simulink model "ivedsp"  (Simulink 7.6)
settings: Solver=FixedStepDiscrete  StartTime=0.0  StopTime=10  FixedStep=1  RelTol=1e-3
libraries: simulink x42
settings Model: Creator=jordan  LastModifiedBy=jordan
settings DataIOCC: LimitDataPoints=off  SaveOutput=off  SignalLogging=off  DSMLogging=off  SaveTime=off
settings OptimizationCC: BlockReduction=off  ConditionallyExecuteInputs=off  InlineParams=on

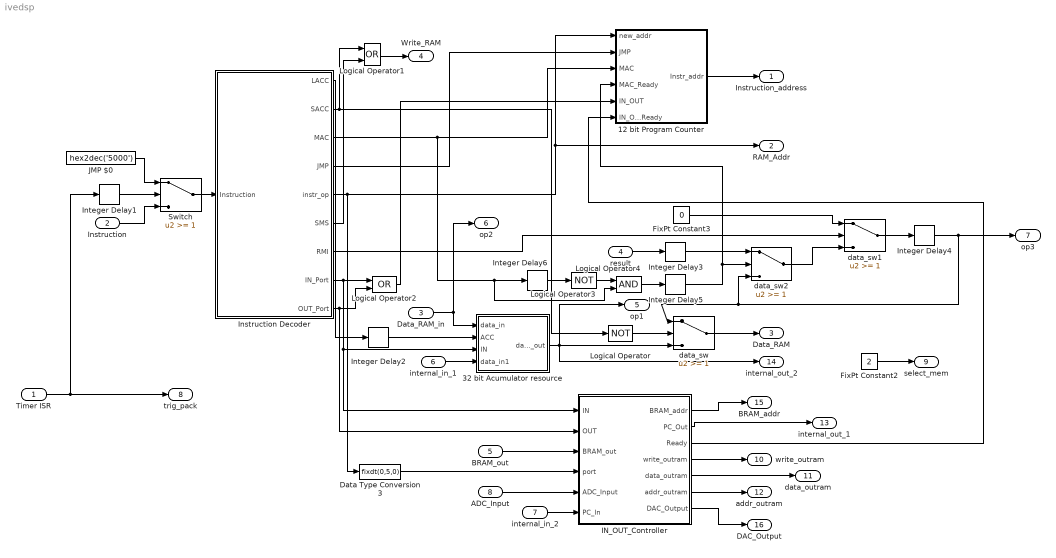
== system ivedsp ==
  Timer ISR : Inport  OutDataTypeStr=boolean
  Instruction : Inport  Port=2  OutDataTypeStr=uint16
  Data_RAM_in : Inport  Port=3  OutDataTypeStr=uint32
  result : Inport  Port=4  OutDataTypeStr=uint32
  BRAM_out : Inport  Port=5  OutDataTypeStr=uint8
  internal_in_1 : Inport  Port=6  OutDataTypeStr=uint32
  internal_in_2 : Inport  Port=7  OutDataTypeStr=uint8  PortDimensions=4
  ADC_Input : Inport  Port=8  OutDataTypeStr=uint8  PortDimensions=8
  12 bit Program Counter : Subsystem
  32 bit Acumulator resource : Subsystem
  Data Type Conversion3 : DataTypeConversion  OutDataTypeStr=fixdt(0,5,0)
  FixPt Constant2 : Constant  DisableCoverage=on  Value=2  OutDataTypeStr=fixdt(0,4,0)
  FixPt Constant3 : Constant  DisableCoverage=on  Value=0  OutDataTypeStr=uint32
  IN_OUT_Controller : Subsystem
  Instruction Decoder : Subsystem
  Integer Delay{1..4,6} (5 alike) : simulink/Discrete/Integer Delay  NumDelays=1  vinit=0.0  samptime=-1
  Integer Delay5 : simulink/Discrete/Integer Delay  NumDelays=3  vinit=0.0  samptime=-1
  JMP $0 : Constant  DisableCoverage=on  Value=hex2dec('5000')  OutDataTypeStr=Inherit: Inherit via back propagation
  Logical Operator : Logic  Operator=NOT  AllPortsSameDT=off  OutDataTypeStr=boolean
  Logical Operator1 : Logic  Operator=OR  AllPortsSameDT=off  OutDataTypeStr=boolean
  Logical Operator2 : Logic  Operator=OR  AllPortsSameDT=off  OutDataTypeStr=boolean
  Logical Operator3 : Logic  Operator=NOT  AllPortsSameDT=off  OutDataTypeStr=boolean
  Logical Operator4 : Logic  AllPortsSameDT=off  OutDataTypeStr=boolean
  Switch : Switch  Threshold=1
  data_sw : Switch  Threshold=1
  data_sw1 : Switch  Threshold=1
  data_sw2 : Switch  Threshold=1
  Instruction_address : Outport  OutDataTypeStr=fixdt(0,12,0)
  RAM_Addr : Outport  Port=2  OutDataTypeStr=fixdt(0,12,0)
  Data_RAM : Outport  Port=3  OutDataTypeStr=uint32
  Write_RAM : Outport  Port=4  OutDataTypeStr=boolean
  op1 : Outport  Port=5  OutDataTypeStr=uint32
  op2 : Outport  Port=6  OutDataTypeStr=uint32
  op3 : Outport  Port=7  OutDataTypeStr=uint32
  trig_pack : Outport  Port=8
  select_mem : Outport  Port=9
  write_outram : Outport  Port=10  OutDataTypeStr=boolean
  data_outram : Outport  Port=11  OutDataTypeStr=uint8
  addr_outram : Outport  Port=12  OutDataTypeStr=fixdt(0,14,0)
  internal_out_1 : Outport  Port=13
  internal_out_2 : Outport  Port=14  OutDataTypeStr=uint32
  BRAM_addr : Outport  Port=15
  DAC_Output : Outport  Port=16
  wires:
  32 bit Acumulator resource/1(data_out) -> data_sw/3, op1/1, internal_out_2/1
  Data_RAM_in/1 -> 32 bit Acumulator resource/1(data_in), op2/1
  Instruction Decoder/5(instr_op) -> 12 bit Program Counter/1(new_addr), RAM_Addr/1, Data Type Conversion3/1
  Instruction Decoder/1(LACC) -> Integer Delay2/1
  Integer Delay2/1 -> 32 bit Acumulator resource/2(ACC)
  Instruction Decoder/2(SACC) -> Logical Operator/1, Logical Operator1/1
  Logical Operator/1 -> data_sw/2
  Instruction Decoder/4(JMP) -> 12 bit Program Counter/2(JMP)
  Instruction Decoder/3(MAC) -> 12 bit Program Counter/3(MAC), Logical Operator4/2, Integer Delay6/1
  Instruction Decoder/7(RMI) -> data_sw1/2
  Instruction Decoder/6(SMS) -> Logical Operator1/2
  Instruction Decoder/8(IN_Port) -> 32 bit Acumulator resource/3(IN), IN_OUT_Controller/1(IN), Logical Operator2/1
  Data Type Conversion3/1 -> IN_OUT_Controller/4(port)
  Switch/1 -> Instruction Decoder/1(Instruction)
  JMP $0/1 -> Switch/1
  12 bit Program Counter/1(Instr_addr) -> Instruction_address/1
  Instruction/1 -> Switch/3
  data_sw/1 -> Data_RAM/1
  Logical Operator1/1 -> Write_RAM/1
  result/1 -> Integer Delay3/1
  Instruction Decoder/9(OUT_Port) -> Logical Operator2/2, IN_OUT_Controller/2(OUT)
  IN_OUT_Controller/6(addr_outram) -> addr_outram/1
  IN_OUT_Controller/4(write_outram) -> write_outram/1
  IN_OUT_Controller/5(data_outram) -> data_outram/1
  Logical Operator2/1 -> 12 bit Program Counter/5(IN_OUT)
  internal_in_1/1 -> 32 bit Acumulator resource/4(data_in1)
  internal_in_2/1 -> IN_OUT_Controller/6(PC_In)
  Integer Delay1/1 -> Switch/2
  FixPt Constant2/1 -> select_mem/1
  Timer ISR/1 -> trig_pack/1, Integer Delay1/1
  Integer Delay4/1 -> op3/1, data_sw2/3, data_sw/1
  data_sw1/1 -> Integer Delay4/1
  FixPt Constant3/1 -> data_sw1/1
  data_sw2/1 -> data_sw1/3
  Integer Delay3/1 -> data_sw2/1
  Integer Delay5/1 -> 12 bit Program Counter/4(MAC_Ready), data_sw2/2
  Integer Delay6/1 -> Logical Operator3/1
  Logical Operator3/1 -> Logical Operator4/1
  Logical Operator4/1 -> Integer Delay5/1
  IN_OUT_Controller/7(DAC_Output) -> DAC_Output/1
  IN_OUT_Controller/3(Ready) -> 12 bit Program Counter/6(IN_OUT_Ready)
  BRAM_out/1 -> IN_OUT_Controller/3(BRAM_out)
  ADC_Input/1 -> IN_OUT_Controller/5(ADC_Input)
  IN_OUT_Controller/2(PC_Out) -> internal_out_1/1
  IN_OUT_Controller/1(BRAM_addr) -> BRAM_addr/1

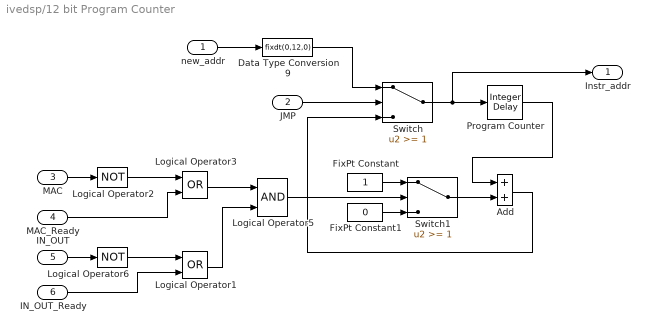
== system ivedsp/12 bit Program Counter ==
  new_addr : Inport
  JMP : Inport  Port=2
  MAC : Inport  Port=3  OutDataTypeStr=boolean
  MAC_Ready : Inport  Port=4  OutDataTypeStr=boolean
  IN_OUT : Inport  Port=5  OutDataTypeStr=boolean
  IN_OUT_Ready : Inport  Port=6  OutDataTypeStr=boolean
  Add : Sum  AccumDataTypeStr=fixdt(0,12,0)  OutDataTypeStr=fixdt(0,12,0)
  Data Type Conversion9 : DataTypeConversion  OutDataTypeStr=fixdt(0,12,0)
  FixPt Constant : Constant  DisableCoverage=on  OutDataTypeStr=fixdt(0,12,0)
  FixPt Constant1 : Constant  DisableCoverage=on  Value=0  OutDataTypeStr=fixdt(0,12,0)
  Logical Operator1 : Logic  Operator=OR  AllPortsSameDT=off  OutDataTypeStr=boolean
  Logical Operator2 : Logic  Operator=NOT  AllPortsSameDT=off  OutDataTypeStr=boolean
  Logical Operator3 : Logic  Operator=OR  AllPortsSameDT=off  OutDataTypeStr=boolean
  Logical Operator5 : Logic  AllPortsSameDT=off  OutDataTypeStr=boolean
  Logical Operator6 : Logic  Operator=NOT  AllPortsSameDT=off  OutDataTypeStr=boolean
  Program Counter : simulink/Discrete/Integer Delay  NumDelays=1  vinit=0.0  samptime=-1
  Switch : Switch  Threshold=1
  Switch1 : Switch  Threshold=1
  Instr_addr : Outport  InitialOutput=0
  wires:
  JMP/1 -> Switch/2
  new_addr/1 -> Data Type Conversion9/1
  Program Counter/1 -> Add/1
  Switch/1 -> Program Counter/1, Instr_addr/1
  FixPt Constant/1 -> Switch1/1
  Add/1 -> Switch/3
  Data Type Conversion9/1 -> Switch/1
  Switch1/1 -> Add/2
  FixPt Constant1/1 -> Switch1/3
  Logical Operator3/1 -> Logical Operator5/1
  Logical Operator2/1 -> Logical Operator3/1
  MAC/1 -> Logical Operator2/1
  Logical Operator1/1 -> Logical Operator5/2
  Logical Operator6/1 -> Logical Operator1/1
  IN_OUT/1 -> Logical Operator6/1
  IN_OUT_Ready/1 -> Logical Operator1/2
  Logical Operator5/1 -> Switch1/2
  MAC_Ready/1 -> Logical Operator3/2

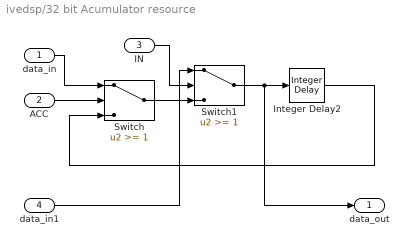
== system ivedsp/32 bit Acumulator resource ==
  data_in : Inport
  ACC : Inport  Port=2
  IN : Inport  Port=3
  data_in1 : Inport  Port=4
  Integer Delay2 : simulink/Discrete/Integer Delay  NumDelays=1  vinit=0.0  samptime=-1
  Switch : Switch  Threshold=1
  Switch1 : Switch  Threshold=1
  data_out : Outport  OutDataTypeStr=uint32
  wires:
  Switch/1 -> Switch1/3
  Integer Delay2/1 -> Switch/3
  data_in/1 -> Switch/1
  ACC/1 -> Switch/2
  Switch1/1 -> Integer Delay2/1, data_out/1
  IN/1 -> Switch1/2
  data_in1/1 -> Switch1/1

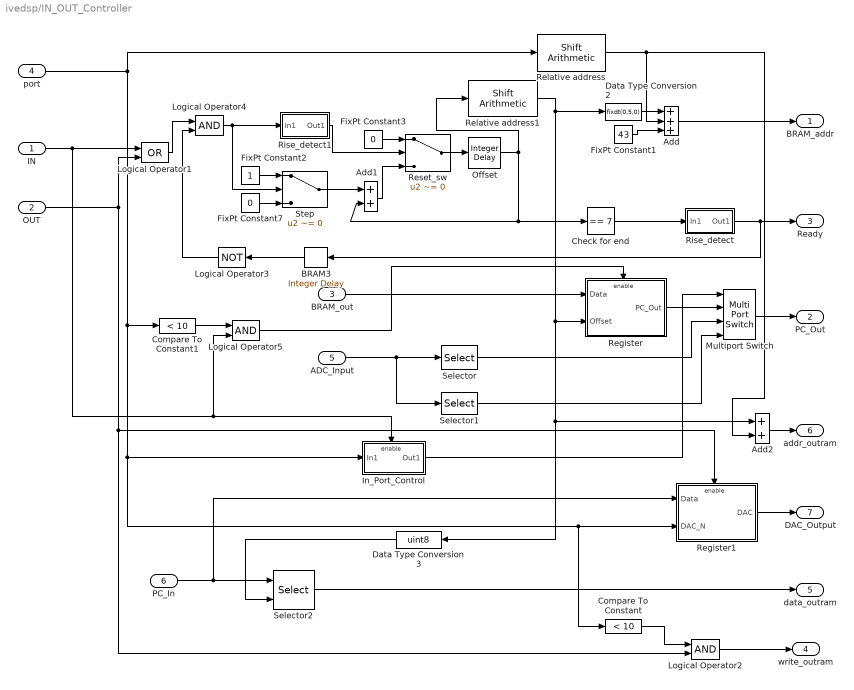
== system ivedsp/IN_OUT_Controller ==
  IN : Inport  OutDataTypeStr=boolean
  OUT : Inport  Port=2  OutDataTypeStr=boolean
  BRAM_out : Inport  Port=3  OutDataTypeStr=uint8
  port : Inport  Port=4  OutDataTypeStr=fixdt(0,5,0)
  ADC_Input : Inport  Port=5  OutDataTypeStr=uint8  PortDimensions=8
  PC_In : Inport  Port=6  OutDataTypeStr=uint8  PortDimensions=4
  Add : Sum  Inputs=+++  AccumDataTypeStr=fixdt(0,11,0)  OutDataTypeStr=fixdt(0,11,0)  SaturateOnIntegerOverflow=on
  Add1 : Sum  AccumDataTypeStr=fixdt(0,3,0)  OutDataTypeStr=fixdt(0,3,0)  SaturateOnIntegerOverflow=on
  Add2 : Sum  AccumDataTypeStr=fixdt(0,14,0)  OutDataTypeStr=fixdt(0,14,0)
  BRAM3 : simulink/Discrete/Integer Delay  NumDelays=1  vinit=0.0  samptime=-1
  Check for end : simulink/Logic and Bit Operations/Compare To Constant  SystemSampleTime=-1  relop===  const=7  LogicOutDataTypeMode=boolean
  Compare To Constant : simulink/Logic and Bit Operations/Compare To Constant  SystemSampleTime=-1  relop=<  const=10  LogicOutDataTypeMode=boolean
  Compare To Constant1 : simulink/Logic and Bit Operations/Compare To Constant  SystemSampleTime=-1  relop=<  const=10  LogicOutDataTypeMode=boolean
  Data Type Conversion2 : DataTypeConversion  OutDataTypeStr=fixdt(0,5,0)
  Data Type Conversion3 : DataTypeConversion  OutDataTypeStr=uint8
  FixPt Constant1 : Constant  DisableCoverage=on  Value=43  OutDataTypeStr=fixdt(0,11,0)
  FixPt Constant2 : Constant  DisableCoverage=on  OutDataTypeStr=fixdt(0,3,0)
  FixPt Constant3 : Constant  DisableCoverage=on  Value=0  OutDataTypeStr=fixdt(0,3,0)
  FixPt Constant7 : Constant  DisableCoverage=on  Value=0  OutDataTypeStr=fixdt(0,3,0)
  In_Port_Control : Subsystem
  Logical Operator1 : Logic  Operator=OR  AllPortsSameDT=off  OutDataTypeStr=boolean
  Logical Operator2 : Logic  AllPortsSameDT=off  OutDataTypeStr=boolean
  Logical Operator3 : Logic  Operator=NOT  AllPortsSameDT=off  OutDataTypeStr=boolean
  Logical Operator4 : Logic  AllPortsSameDT=off  OutDataTypeStr=boolean
  Logical Operator5 : Logic  AllPortsSameDT=off  OutDataTypeStr=boolean
  Multiport Switch : MultiPortSwitch  DataPortOrder=Zero-based contiguous  zeroidx=on
  Offset : simulink/Discrete/Integer Delay  NumDelays=1  vinit=0.0  samptime=0
  Register : Subsystem
  Register1 : Subsystem
  Relative address : simulink/Logic and Bit Operations/Shift Arithmetic  SystemSampleTime=-1  nBitShiftRight=-2  nBinPtShiftRight=0
  Relative address1 : simulink/Logic and Bit Operations/Shift Arithmetic  SystemSampleTime=-1  nBitShiftRight=1  nBinPtShiftRight=0
  Reset_sw : Switch  Criteria=u2 ~= 0
  Rise_detect : Subsystem
  Rise_detect1 : Subsystem
  Selector : Selector  InputPortWidth=8  IndexOptions=Index vector (dialog)  Indices=1:4  OutputSizes=1
  Selector1 : Selector  InputPortWidth=8  IndexOptions=Index vector (dialog)  Indices=5:8  OutputSizes=1
  Selector2 : Selector  IndexMode=Zero-based  InputPortWidth=4  IndexOptions=Index vector (port)  Indices=5:8  OutputSizes=1
  Step : Switch  Criteria=u2 ~= 0
  BRAM_addr : Outport
  PC_Out : Outport  Port=2  OutDataTypeStr=uint8  PortDimensions=4
  Ready : Outport  Port=3
  write_outram : Outport  Port=4
  data_outram : Outport  Port=5
  addr_outram : Outport  Port=6
  DAC_Output : Outport  Port=7  OutDataTypeStr=uint8  PortDimensions=8
  wires:
  Register1/1(DAC) -> DAC_Output/1
  OUT/1 -> Logical Operator1/2, Logical Operator2/2, Register1/Enable
  IN/1 -> Logical Operator1/1, In_Port_Control/Enable, Logical Operator5/2
  Selector2/1 -> data_outram/1
  PC_In/1 -> Selector2/1, Register1/1(Data)
  Add2/1 -> addr_outram/1
  BRAM_out/1 -> Register/1(Data)
  FixPt Constant7/1 -> Step/3
  Step/1 -> Add1/1
  In_Port_Control/1(Out1) -> Multiport Switch/1
  Selector1/1 -> Multiport Switch/4
  ADC_Input/1 -> Selector1/1, Selector/1
  Selector/1 -> Multiport Switch/3
  Multiport Switch/1 -> PC_Out/1
  Check for end/1 -> Rise_detect/1(In1)
  FixPt Constant3/1 -> Reset_sw/1
  Rise_detect1/1(Out1) -> Reset_sw/2
  Register/1(PC_Out) -> Multiport Switch/2
  Logical Operator4/1 -> Rise_detect1/1(In1), Step/2
  port/1 -> Relative address/1, In_Port_Control/1(In1), Register1/2(DAC_N), Compare To Constant/1, Compare To Constant1/1
  Relative address/1 -> Add2/2, Add/2
  FixPt Constant2/1 -> Step/1
  Add1/1 -> Reset_sw/3
  Reset_sw/1 -> Offset/1
  FixPt Constant1/1 -> Add/3
  Data Type Conversion2/1 -> Add/1
  Add/1 -> BRAM_addr/1
  Offset/1 -> Relative address1/1, Add1/2, Check for end/1
  Rise_detect/1(Out1) -> Ready/1, BRAM3/1
  Data Type Conversion3/1 -> Selector2/2
  Relative address1/1 -> Data Type Conversion2/1, Register/2(Offset), Add2/1, Data Type Conversion3/1
  Logical Operator2/1 -> write_outram/1
  Compare To Constant/1 -> Logical Operator2/1
  Logical Operator3/1 -> Logical Operator4/2
  Logical Operator1/1 -> Logical Operator4/1
  BRAM3/1 -> Logical Operator3/1
  Logical Operator5/1 -> Register/Enable
  Compare To Constant1/1 -> Logical Operator5/1

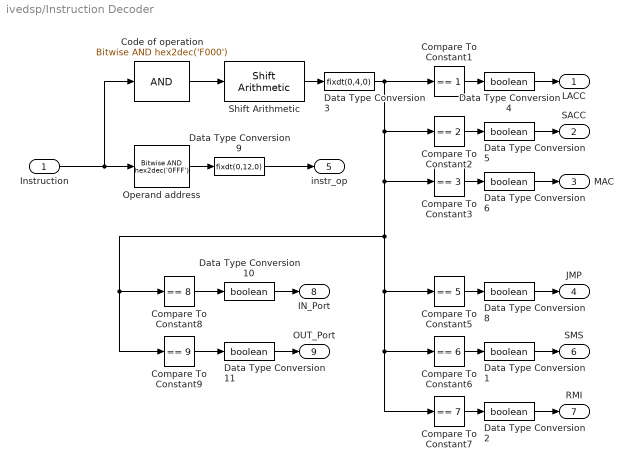
== system ivedsp/Instruction Decoder ==
  Instruction : Inport  OutDataTypeStr=uint16
  Code of operation : simulink/Logic and Bit Operations/Bitwise Operator  logicop=AND  UseBitMask=on  BitMask=hex2dec('F000')  BitMaskRealWorld=Stored Integer
  Compare To Constant1 : simulink/Logic and Bit Operations/Compare To Constant  SystemSampleTime=-1  relop===  const=1  LogicOutDataTypeMode=boolean
  Compare To Constant2 : simulink/Logic and Bit Operations/Compare To Constant  SystemSampleTime=-1  relop===  const=2  LogicOutDataTypeMode=boolean
  Compare To Constant3 : simulink/Logic and Bit Operations/Compare To Constant  SystemSampleTime=-1  relop===  const=3  LogicOutDataTypeMode=boolean
  Compare To Constant5 : simulink/Logic and Bit Operations/Compare To Constant  SystemSampleTime=-1  relop===  const=5  LogicOutDataTypeMode=boolean
  Compare To Constant6 : simulink/Logic and Bit Operations/Compare To Constant  SystemSampleTime=-1  relop===  const=6  LogicOutDataTypeMode=boolean
  Compare To Constant7 : simulink/Logic and Bit Operations/Compare To Constant  SystemSampleTime=-1  relop===  const=7  LogicOutDataTypeMode=boolean
  Compare To Constant8 : simulink/Logic and Bit Operations/Compare To Constant  SystemSampleTime=-1  relop===  const=8  LogicOutDataTypeMode=boolean
  Compare To Constant9 : simulink/Logic and Bit Operations/Compare To Constant  SystemSampleTime=-1  relop===  const=9  LogicOutDataTypeMode=boolean
  Data Type Conversion{1..2,4..6,8,10..11} (8 alike) : DataTypeConversion  OutDataTypeStr=boolean
  Data Type Conversion3 : DataTypeConversion  OutDataTypeStr=fixdt(0,4,0)
  Data Type Conversion9 : DataTypeConversion  OutDataTypeStr=fixdt(0,12,0)
  Operand address : simulink/Logic and Bit Operations/Bitwise Operator  logicop=AND  UseBitMask=on  BitMask=hex2dec('0FFF')  BitMaskRealWorld=Stored Integer
  Shift Arithmetic : simulink/Logic and Bit Operations/Shift Arithmetic  SystemSampleTime=-1  nBitShiftRight=12  nBinPtShiftRight=0
  LACC : Outport
  SACC : Outport  Port=2
  MAC : Outport  Port=3
  JMP : Outport  Port=4
  instr_op : Outport  Port=5
  SMS : Outport  Port=6
  RMI : Outport  Port=7
  IN_Port : Outport  Port=8
  OUT_Port : Outport  Port=9
  wires:
  Instruction/1 -> Operand address/1, Code of operation/1
  Code of operation/1 -> Shift Arithmetic/1
  Shift Arithmetic/1 -> Data Type Conversion3/1
  Data Type Conversion3/1 -> Compare To Constant6/1, Compare To Constant7/1, Compare To Constant5/1, Compare To Constant8/1, Compare To Constant9/1, Compare To Constant3/1, Compare To Constant2/1, Compare To Constant1/1
  Compare To Constant1/1 -> Data Type Conversion4/1
  Compare To Constant2/1 -> Data Type Conversion5/1
  Compare To Constant3/1 -> Data Type Conversion6/1
  Compare To Constant5/1 -> Data Type Conversion8/1
  Operand address/1 -> Data Type Conversion9/1
  Data Type Conversion4/1 -> LACC/1
  Data Type Conversion5/1 -> SACC/1
  Data Type Conversion9/1 -> instr_op/1
  Data Type Conversion6/1 -> MAC/1
  Data Type Conversion8/1 -> JMP/1
  Compare To Constant6/1 -> Data Type Conversion1/1
  Data Type Conversion1/1 -> SMS/1
  Compare To Constant7/1 -> Data Type Conversion2/1
  Data Type Conversion2/1 -> RMI/1
  Compare To Constant8/1 -> Data Type Conversion10/1
  Data Type Conversion10/1 -> IN_Port/1
  Compare To Constant9/1 -> Data Type Conversion11/1
  Data Type Conversion11/1 -> OUT_Port/1

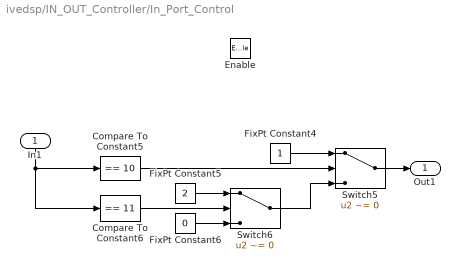
== system ivedsp/IN_OUT_Controller/In_Port_Control ==
  In1 : Inport
  Enable : EnablePort
  Compare To Constant5 : simulink/Logic and Bit Operations/Compare To Constant  SystemSampleTime=-1  relop===  const=10  LogicOutDataTypeMode=boolean
  Compare To Constant6 : simulink/Logic and Bit Operations/Compare To Constant  SystemSampleTime=-1  relop===  const=11  LogicOutDataTypeMode=boolean
  FixPt Constant4 : Constant  DisableCoverage=on  OutDataTypeStr=fixdt(0,2,0)
  FixPt Constant5 : Constant  DisableCoverage=on  Value=2  OutDataTypeStr=fixdt(0,2,0)
  FixPt Constant6 : Constant  DisableCoverage=on  Value=0  OutDataTypeStr=fixdt(0,2,0)
  Switch5 : Switch  Criteria=u2 ~= 0
  Switch6 : Switch  Criteria=u2 ~= 0
  Out1 : Outport  InitialOutput=0
  wires:
  Switch6/1 -> Switch5/3
  FixPt Constant6/1 -> Switch6/3
  FixPt Constant5/1 -> Switch6/1
  FixPt Constant4/1 -> Switch5/1
  Compare To Constant6/1 -> Switch6/2
  Compare To Constant5/1 -> Switch5/2
  In1/1 -> Compare To Constant6/1, Compare To Constant5/1
  Switch5/1 -> Out1/1

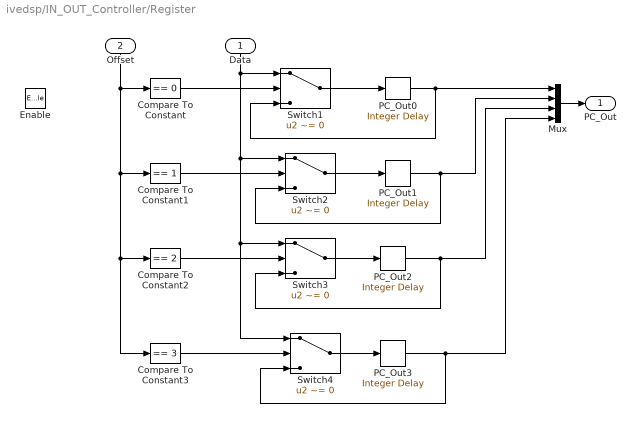
== system ivedsp/IN_OUT_Controller/Register ==
  Data : Inport
  Offset : Inport  Port=2
  Enable : EnablePort
  Compare To Constant : simulink/Logic and Bit Operations/Compare To Constant  SystemSampleTime=-1  relop===  const=0  LogicOutDataTypeMode=boolean
  Compare To Constant1 : simulink/Logic and Bit Operations/Compare To Constant  SystemSampleTime=-1  relop===  const=1  LogicOutDataTypeMode=boolean
  Compare To Constant2 : simulink/Logic and Bit Operations/Compare To Constant  SystemSampleTime=-1  relop===  const=2  LogicOutDataTypeMode=boolean
  Compare To Constant3 : simulink/Logic and Bit Operations/Compare To Constant  SystemSampleTime=-1  relop===  const=3  LogicOutDataTypeMode=boolean
  Mux : Mux
  PC_Out{0..3} (4 alike) : simulink/Discrete/Integer Delay  NumDelays=1  vinit=0.0  samptime=-1
  Switch{1..4} (4 alike) : Switch  Criteria=u2 ~= 0
  PC_Out : Outport  InitialOutput=0
  wires:
  Mux/1 -> PC_Out/1
  Offset/1 -> Compare To Constant1/1, Compare To Constant3/1, Compare To Constant2/1, Compare To Constant/1
  Data/1 -> Switch4/1, Switch3/1, Switch2/1, Switch1/1
  Compare To Constant3/1 -> Switch4/2
  PC_Out3/1 -> Mux/4, Switch4/3
  Switch4/1 -> PC_Out3/1
  Compare To Constant2/1 -> Switch3/2
  PC_Out2/1 -> Mux/3, Switch3/3
  Switch3/1 -> PC_Out2/1
  Compare To Constant1/1 -> Switch2/2
  PC_Out1/1 -> Mux/2, Switch2/3
  Switch2/1 -> PC_Out1/1
  Compare To Constant/1 -> Switch1/2
  PC_Out0/1 -> Mux/1, Switch1/3
  Switch1/1 -> PC_Out0/1

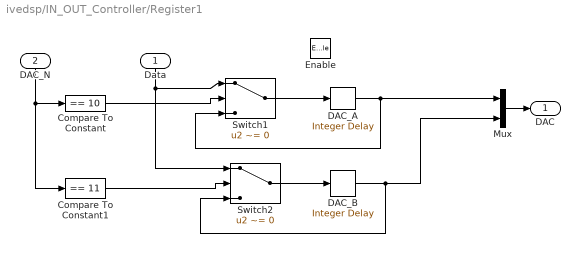
== system ivedsp/IN_OUT_Controller/Register1 ==
  Data : Inport
  DAC_N : Inport  Port=2
  Enable : EnablePort
  Compare To Constant : simulink/Logic and Bit Operations/Compare To Constant  SystemSampleTime=-1  relop===  const=10  LogicOutDataTypeMode=boolean
  Compare To Constant1 : simulink/Logic and Bit Operations/Compare To Constant  SystemSampleTime=-1  relop===  const=11  LogicOutDataTypeMode=boolean
  DAC_A : simulink/Discrete/Integer Delay  NumDelays=1  vinit=0.0  samptime=-1
  DAC_B : simulink/Discrete/Integer Delay  NumDelays=1  vinit=0.0  samptime=-1
  Mux : Mux  Inputs=2
  Switch1 : Switch  Criteria=u2 ~= 0
  Switch2 : Switch  Criteria=u2 ~= 0
  DAC : Outport  InitialOutput=0
  wires:
  Switch1/1 -> DAC_A/1
  DAC_A/1 -> Switch1/3, Mux/1
  Compare To Constant/1 -> Switch1/2
  Switch2/1 -> DAC_B/1
  DAC_B/1 -> Switch2/3, Mux/2
  Compare To Constant1/1 -> Switch2/2
  Data/1 -> Switch1/1, Switch2/1
  DAC_N/1 -> Compare To Constant/1, Compare To Constant1/1
  Mux/1 -> DAC/1

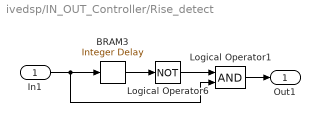
== system ivedsp/IN_OUT_Controller/Rise_detect ==
  In1 : Inport
  BRAM3 : simulink/Discrete/Integer Delay  NumDelays=1  vinit=0.0  samptime=-1
  Logical Operator1 : Logic  AllPortsSameDT=off  OutDataTypeStr=boolean
  Logical Operator6 : Logic  Operator=NOT  AllPortsSameDT=off  OutDataTypeStr=boolean
  Out1 : Outport
  wires:
  Logical Operator1/1 -> Out1/1
  In1/1 -> Logical Operator1/2, BRAM3/1
  BRAM3/1 -> Logical Operator6/1
  Logical Operator6/1 -> Logical Operator1/1

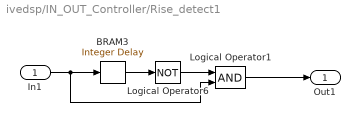
== system ivedsp/IN_OUT_Controller/Rise_detect1 ==
  In1 : Inport
  BRAM3 : simulink/Discrete/Integer Delay  NumDelays=1  vinit=0.0  samptime=-1
  Logical Operator1 : Logic  AllPortsSameDT=off  OutDataTypeStr=boolean
  Logical Operator6 : Logic  Operator=NOT  AllPortsSameDT=off  OutDataTypeStr=boolean
  Out1 : Outport
  wires:
  Logical Operator6/1 -> Logical Operator1/1
  BRAM3/1 -> Logical Operator6/1
  In1/1 -> BRAM3/1, Logical Operator1/2
  Logical Operator1/1 -> Out1/1
